simulink model "PowerGenSim"  (R2024b)
settings: Solver=VariableStepAuto  StartTime=0.0  StopTime=sat.T  RelTol=1e-3
values from neighbouring files (symbols this model uses):
  Re = 6378e03    (= 6378000)    [PowerGenSim_Params.m]
undefined symbols (not defined in the file or in its folder): sat
libraries: vrlib x4, matrix_library x2, simulink_extras x1
settings Model: Creator=Ameya  LastModifiedBy=Ameya

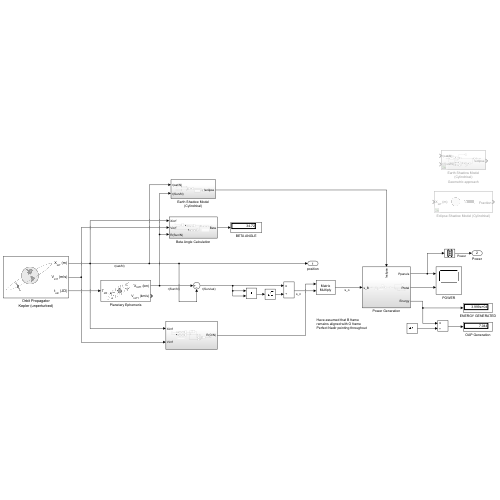
[thumbnail: Simulink's stored preview of the top-level diagram]
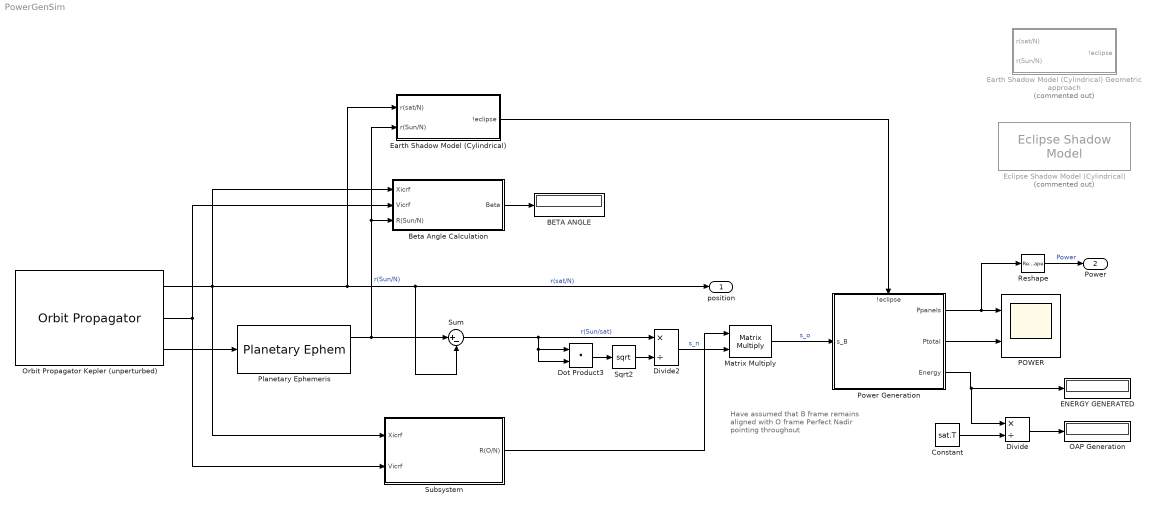
== system PowerGenSim ==
  note: Have assumed that B frame remains aligned with O frame
      | Perfect Nadir pointing throughout
  BETA ANGLE : Display
  Beta Angle Calculation : Subsystem
  Constant : Constant  Value=sat.T
  Divide : Product  Inputs=*/
  Divide2 : Product  Inputs=*/
  Dot Product3 : DotProduct  OutDataTypeStr=Inherit: Inherit via internal rule
  ENERGY GENERATED : Display
  Earth Shadow Model (Cylindrical) : Subsystem
  Earth Shadow Model (Cylindrical) Geometric approach : Subsystem  Commented=on
  Eclipse Shadow Model (Cylindrical) : EclipseShadowModel  Commented=on  shadowModel=Cylindrical  startDate=initialTimeJD  includeMoon=off  useEphemerisDateRange=off
  Matrix Multiply : Product  Multiplication=Matrix(*)
  OAP Generation : Display
  Orbit Propagator Kepler (unperturbed) : OrbitPropagator  startDate=initialTimeJD  semiMajorAxis=sat.a  eccentricity=sat.e  inclination=sat.i  raan=sat.RAAN  argPeriapsis=sat.w  trueAnomaly=sat.f  inertialPosition=[3649700.0 3308200.0 -4676600.0]  inertialVelocity=[-2750.8 6666.4 2573.4]  fixedPosition=[-4142689.0 -2676864.7 -4669861.6]  fixedVelocity=[1452.7 -6720.7 2568.1]  customR=3396200  customMu=4.305e13  customJ2=1.0826269e-03  customOmega=4.06125949e-3
  POWER : Scope  NumInputPorts=2
  Planetary Ephemeris : PlanetaryEphem  target=Sun
  Power Generation : Subsystem
      settings: PortSchema="{\"entries\":[{\"content\":{\"sides\":[{\"content\":{\"connectorIds\":[\"In1\"]},\"type\":\"ConnectorPlacement.EquallySpacedRectSide\",\"uuid\":\"8d446733-69e8-48a0-ae35-006265559fdb\"},{\"content\":{\"connectorIds\":[\"Out1\",\"Out2\",\"Out3\"],\"side\":\"RIGHT\"},\"type\":\"ConnectorPlacement.EquallySpacedRectSide\",\"uuid\":\"081b3f49-1ee9-4aa1-bea1-61239cdc4507\"},{\"content\":{\"connectorIds\":[\"In2\"],\"side\":\"TOP\"},\"type\":\"ConnectorPlacement.EquallySpacedRectSide\",\"uuid\":\"b68fd0b1-c1d0-4a3a-b207-adf3131eec8b\"}]},\"type\":\"ConnectorPlacement.EquallySpacedConnector\",\"uuid\":\"c5f8928d-ef3b-4c68-b6c6-8ab80b1a820a\"}],\"packageUris\":[\"http://schema.mathworks.com/mf0/Connector/R2020b\"],\"version\":\"1.0\"}"
  Reshape : Reshape  OutputDimensionality=Column vector (2-D)
  Sqrt2 : Sqrt
  Subsystem : Subsystem
  Sum : Sum  Inputs=|+-
  position : Outport
  Power : Outport  Port=2
  wires:
  Orbit Propagator Kepler (unperturbed)/1 -> Beta Angle Calculation/1(Xicrf), Earth Shadow Model (Cylindrical)/1(r(sat/N)), position/1, Sum/2, Subsystem/1(Xicrf)  "r(sat/N)"
  Orbit Propagator Kepler (unperturbed)/3 -> Planetary Ephemeris/1
  Planetary Ephemeris/1 -> Earth Shadow Model (Cylindrical)/2(r(Sun/N)), Beta Angle Calculation/3(R(Sun/N)), Sum/1  "r(Sun/N)"
  Sqrt2/1 -> Divide2/2
  Dot Product3/1 -> Sqrt2/1
  Divide2/1 -> Matrix Multiply/2  "s_n"
  Subsystem/1(R(O/N)) -> Matrix Multiply/1
  Orbit Propagator Kepler (unperturbed)/2 -> Beta Angle Calculation/2(Vicrf), Subsystem/2(Vicrf)
  Sum/1 -> Dot Product3/2, Dot Product3/1, Divide2/1  "r(Sun/sat)"
  Matrix Multiply/1 -> Power Generation/1(s_B)  "s_o"
  Power Generation/1(Ppanels) -> Reshape/1, POWER/1
  Power Generation/2(Ptotal) -> POWER/2
  Power Generation/3(Energy) -> Divide/1, ENERGY GENERATED/1
  Beta Angle Calculation/1(Beta) -> BETA ANGLE/1
  Earth Shadow Model (Cylindrical)/1(!eclipse) -> Power Generation/2(!eclipse)
  Constant/1 -> Divide/2
  Divide/1 -> OAP Generation/1
  Reshape/1 -> Power/1  "Power"

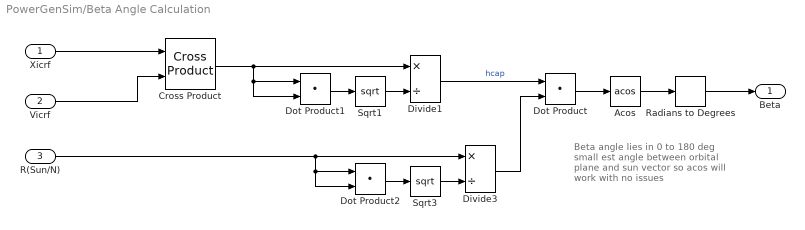
== system PowerGenSim/Beta Angle Calculation ==
  note: Beta angle lies in 0 to 180 deg
      | small est angle between orbital plane and sun vector
      | so acos will work with no issues
  Xicrf : Inport
  Vicrf : Inport  Port=2
  R(Sun/N) : Inport  Port=3
  Acos : Trigonometry  Operator=acos
  Cross Product : matrix_library/Cross Product
  Divide1 : Product  Inputs=*/
  Divide3 : Product  Inputs=*/
  Dot Product : DotProduct  OutDataTypeStr=Inherit: Inherit via internal rule
  Dot Product1 : DotProduct  OutDataTypeStr=Inherit: Inherit via internal rule
  Dot Product2 : DotProduct  OutDataTypeStr=Inherit: Inherit via internal rule
  Radians to Degrees : simulink_extras/Transformations/Radians to Degrees
  Sqrt1 : Sqrt
  Sqrt3 : Sqrt
  Beta : Outport
  wires:
  Divide3/1 -> Dot Product/2
  Sqrt3/1 -> Divide3/2
  Dot Product/1 -> Acos/1
  Dot Product2/1 -> Sqrt3/1
  Cross Product/1 -> Dot Product1/1, Dot Product1/2, Divide1/1
  Acos/1 -> Radians to Degrees/1
  R(Sun/N)/1 -> Dot Product2/2, Dot Product2/1, Divide3/1
  Divide1/1 -> Dot Product/1  "hcap"
  Sqrt1/1 -> Divide1/2
  Dot Product1/1 -> Sqrt1/1
  Vicrf/1 -> Cross Product/2
  Radians to Degrees/1 -> Beta/1
  Xicrf/1 -> Cross Product/1

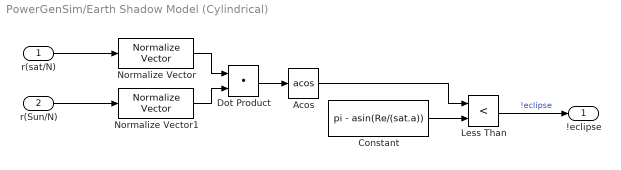
== system PowerGenSim/Earth Shadow Model (Cylindrical) ==
  r(sat/N) : Inport
  r(Sun/N) : Inport  Port=2
  Acos : Trigonometry  Operator=acos
  Constant : Constant  Value=pi - asin(Re/(sat.a))
  Dot Product : DotProduct  OutDataTypeStr=Inherit: Inherit via internal rule
  Less Than : RelationalOperator  Operator=<  OutDataTypeStr=boolean  RndMeth=Simplest  InputSameDT=off
  Normalize Vector : vrlib/Utilities/Normalize Vector  maxzero=0
  Normalize Vector1 : vrlib/Utilities/Normalize Vector  maxzero=0
  !eclipse : Outport
  wires:
  Constant/1 -> Less Than/2
  r(sat/N)/1 -> Normalize Vector/1
  Less Than/1 -> !eclipse/1  "!eclipse"
  Normalize Vector/1 -> Dot Product/1
  Normalize Vector1/1 -> Dot Product/2
  Dot Product/1 -> Acos/1
  Acos/1 -> Less Than/1
  r(Sun/N)/1 -> Normalize Vector1/1

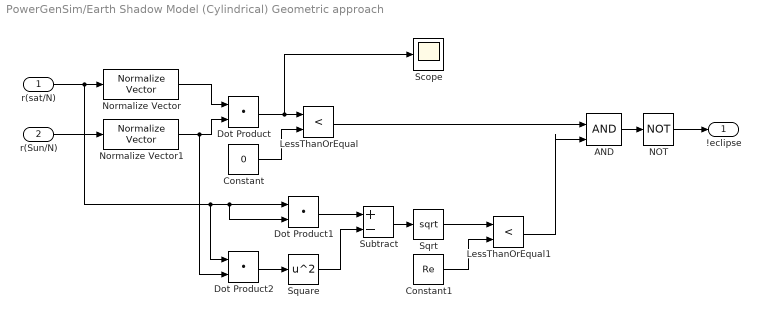
== system PowerGenSim/Earth Shadow Model (Cylindrical) Geometric approach ==
  r(sat/N) : Inport
  r(Sun/N) : Inport  Port=2
  AND : Logic  IconShape=distinctive  AllPortsSameDT=off  OutDataTypeStr=boolean
  Constant : Constant  Value=0
  Constant1 : Constant  Value=Re
  Dot Product : DotProduct  OutDataTypeStr=Inherit: Inherit via internal rule
  Dot Product1 : DotProduct  OutDataTypeStr=Inherit: Inherit via internal rule
  Dot Product2 : DotProduct  OutDataTypeStr=Inherit: Inherit via internal rule
  LessThanOrEqual : RelationalOperator  Operator=<  OutDataTypeStr=boolean  RndMeth=Simplest  InputSameDT=off
  LessThanOrEqual1 : RelationalOperator  Operator=<  OutDataTypeStr=boolean  RndMeth=Simplest  InputSameDT=off
  NOT : Logic  Operator=NOT  IconShape=distinctive  AllPortsSameDT=off  OutDataTypeStr=boolean
  Normalize Vector : vrlib/Utilities/Normalize Vector  maxzero=0
  Normalize Vector1 : vrlib/Utilities/Normalize Vector  maxzero=0
  Scope : Scope
  Sqrt : Sqrt
  Square : Math  Operator=square
  Subtract : Sum  Inputs=+-
  !eclipse : Outport
  wires:
  r(sat/N)/1 -> Dot Product1/2, Dot Product1/1, Dot Product2/1, Normalize Vector/1
  Normalize Vector/1 -> Dot Product/1
  Normalize Vector1/1 -> Dot Product/2, Dot Product2/2
  Dot Product/1 -> Scope/1, LessThanOrEqual/1
  r(Sun/N)/1 -> Normalize Vector1/1
  Constant/1 -> LessThanOrEqual/2
  Dot Product1/1 -> Subtract/1
  Square/1 -> Subtract/2
  Subtract/1 -> Sqrt/1
  Sqrt/1 -> LessThanOrEqual1/1
  Constant1/1 -> LessThanOrEqual1/2
  LessThanOrEqual/1 -> AND/1
  LessThanOrEqual1/1 -> AND/2
  AND/1 -> NOT/1
  Dot Product2/1 -> Square/1
  NOT/1 -> !eclipse/1

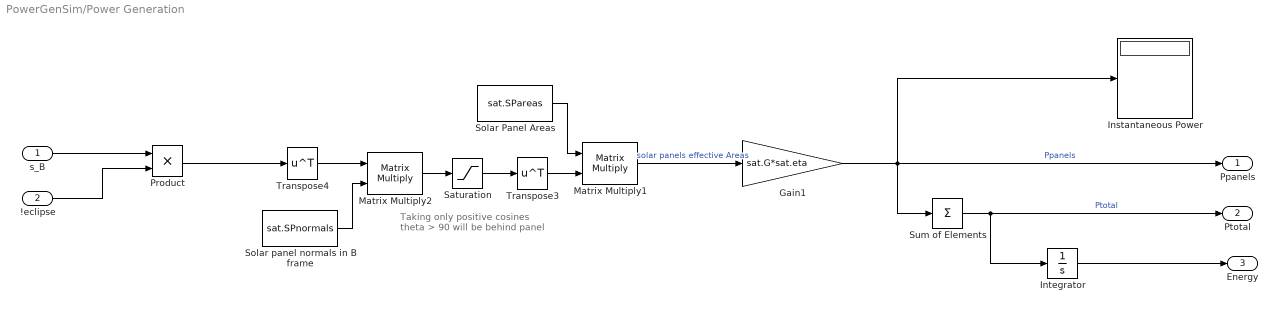
== system PowerGenSim/Power Generation ==
  note: Taking only positive cosines
      | theta > 90 will be behind panel
  s_B : Inport
  !eclipse : Inport  Port=2
  Gain1 : Gain  Gain=sat.G*sat.eta
  Instantaneous Power : Display
  Integrator : Integrator
  Matrix Multiply1 : Product  Multiplication=Matrix(*)
  Matrix Multiply2 : Product  Multiplication=Matrix(*)
  Product : Product
  Saturation : Saturate  UpperLimit=inf  LowerLimit=0
  Solar Panel Areas : Constant  Value=sat.SPareas
  Solar panel normals in B frame : Constant  Value=sat.SPnormals
  Sum of Elements : Sum  Inputs=+
  Transpose3 : Math  Operator=transpose
  Transpose4 : Math  Operator=transpose
  Ppanels : Outport
  Ptotal : Outport  Port=2
  Energy : Outport  Port=3
  wires:
  Saturation/1 -> Transpose3/1
  Sum of Elements/1 -> Ptotal/1, Integrator/1  "Ptotal"
  Matrix Multiply1/1 -> Gain1/1  "solar panels effective Areas"
  Transpose3/1 -> Matrix Multiply1/2
  Gain1/1 -> Ppanels/1, Sum of Elements/1, Instantaneous Power/1  "Ppanels"
  Transpose4/1 -> Matrix Multiply2/1
  s_B/1 -> Product/1
  Solar panel normals in B frame/1 -> Matrix Multiply2/2
  Solar Panel Areas/1 -> Matrix Multiply1/1
  Matrix Multiply2/1 -> Saturation/1
  Integrator/1 -> Energy/1
  Product/1 -> Transpose4/1
  !eclipse/1 -> Product/2

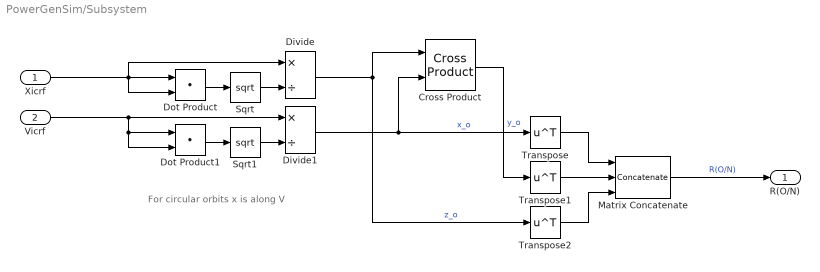
== system PowerGenSim/Subsystem ==
  note: For circular orbits x is along V
  Xicrf : Inport
  Vicrf : Inport  Port=2
  Cross Product : matrix_library/Cross Product
  Divide : Product  Inputs=*/
  Divide1 : Product  Inputs=*/
  Dot Product : DotProduct  OutDataTypeStr=Inherit: Inherit via internal rule
  Dot Product1 : DotProduct  OutDataTypeStr=Inherit: Inherit via internal rule
  Matrix Concatenate : Concatenate  NumInputs=3  Mode=Multidimensional array
  Sqrt : Sqrt
  Sqrt1 : Sqrt
  Transpose : Math  Operator=transpose
  Transpose1 : Math  Operator=transpose
  Transpose2 : Math  Operator=transpose
  R(O/N) : Outport
  wires:
  Transpose2/1 -> Matrix Concatenate/3
  Dot Product/1 -> Sqrt/1
  Vicrf/1 -> Dot Product1/1, Dot Product1/2, Divide1/1
  Divide1/1 -> Transpose/1, Cross Product/2  "x_o"
  Xicrf/1 -> Divide/1, Dot Product/1, Dot Product/2
  Transpose/1 -> Matrix Concatenate/1
  Cross Product/1 -> Transpose1/1  "y_o"
  Divide/1 -> Transpose2/1, Cross Product/1  "z_o"
  Sqrt/1 -> Divide/2
  Sqrt1/1 -> Divide1/2
  Dot Product1/1 -> Sqrt1/1
  Transpose1/1 -> Matrix Concatenate/2
  Matrix Concatenate/1 -> R(O/N)/1  "R(O/N)"
